simulink model "Stability_model"  (R2023a)
settings: Solver=VariableStepAuto  StartTime=0.0  StopTime=600  RelTol=1e-3
libraries: SignalEditorBlockLib x1
settings Model: Creator=levir  LastModifiedBy=levir

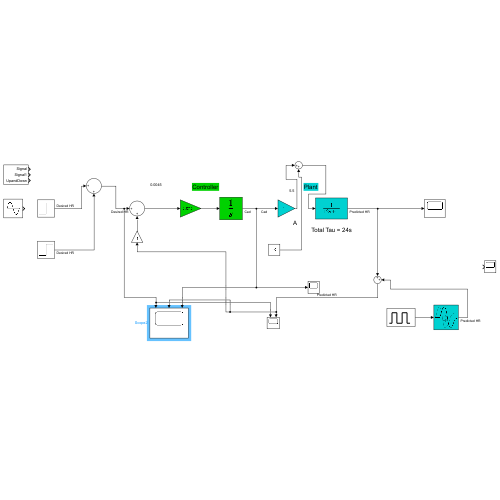
[thumbnail: Simulink's stored preview of the top-level diagram]
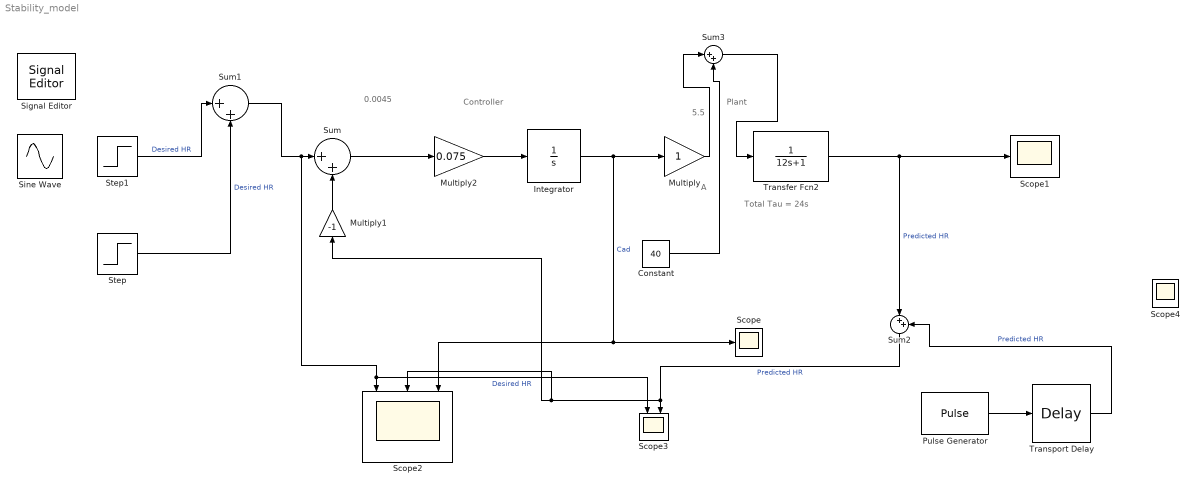
== system Stability_model ==
  note: 5.5
  note: 0.0045
  note: Total Tau = 24s
  note: A
  note: Controller
  note: Plant
  Constant : Constant  Value=40
  Integrator : Integrator
  Multiply : Gain
  Multiply1 : Gain  Gain=-1
  Multiply2 : Gain  Gain=0.075
  Pulse Generator : DiscretePulseGenerator  PulseType=Time based  Amplitude=0  Period=3000
  Scope : Scope
  Scope1 : Scope
  Scope2 : Scope  NumInputPorts=3
  Scope3 : Scope  NumInputPorts=2
  Scope4 : Scope
  Signal Editor : SignalEditorBlockLib/Signal Editor  FileName=C:\Users\levir\OneDrive\Documents\MATLAB\Thesis\testingWave.mat  ActiveScenario=Scenario  ActiveSignal=Signal  IsBus=off  OutputBusObjectStr=Bus: BusObject  SampleTime=0  Interpolate=off  ZeroCross=off  OutputAfterFinalValue=Setting to zero  Unit=inherit  PreserveSignalName=on  ApplySigPropsToAllScenarios=on
  Sine Wave : Sin  Amplitude=20  Bias=140  Frequency=0.05  SampleTime=0
  Step : Step  Time=300  After=50  SampleTime=0
  Step1 : Step  Time=0  Before=60  After=130  SampleTime=0
  Sum{,1..3} (4 alike) : Sum  Inputs=|++
  Transfer Fcn2 : TransferFcn  Denominator=[12 1]
  Transport Delay : TransportDelay  DelayTime=200
  wires:
  Sum/1 -> Multiply2/1
  Multiply2/1 -> Integrator/1
  Transfer Fcn2/1 -> Sum2/1, Scope1/1  "Predicted HR"
  Integrator/1 -> Multiply/1, Scope/1, Scope2/3  "Cad"
  Multiply1/1 -> Sum/2
  Step1/1 -> Sum1/1  "Desired HR"
  Multiply/1 -> Sum3/1
  Step/1 -> Sum1/2  "Desired HR"
  Sum1/1 -> Scope3/1, Scope2/1, Sum/1  "Desired HR"
  Pulse Generator/1 -> Transport Delay/1
  Transport Delay/1 -> Sum2/2  "Predicted HR"
  Sum2/1 -> Scope2/2, Multiply1/1, Scope3/2  "Predicted HR"
  Constant/1 -> Sum3/2
  Sum3/1 -> Transfer Fcn2/1
